simulink model "halfCar_Body"  (R2023b)
settings: Solver=VariableStepAuto  StartTime=0.0  StopTime=10.0  RelTol=1e-3
values from neighbouring files (symbols this model uses):
  a = 1.35    [Parameters.m]
  b = 1.5    [Parameters.m]
  g = 9.81    [Parameters.m]
  I = 650    [Parameters.m]
undefined symbols (not defined in the file or in its folder): Ff, Fr, mb
libraries: simulink x4
settings Model: Creator=crs59  LastModifiedBy=franc
settings DebuggingCC: UnconnectedInputMsg=warning  UnconnectedOutputMsg=warning  UnconnectedLineMsg=warning
settings ModelReferenceCC: EnableRefExpFcnMdlSchedulingChecks=on
settings RTWCC: DLArmComputeVersion=19.05

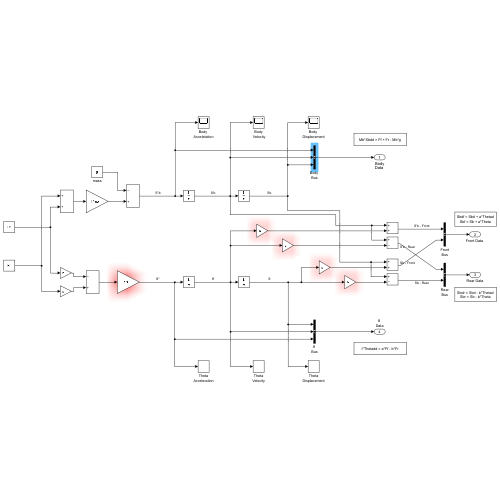
[thumbnail: Simulink's stored preview of the top-level diagram]
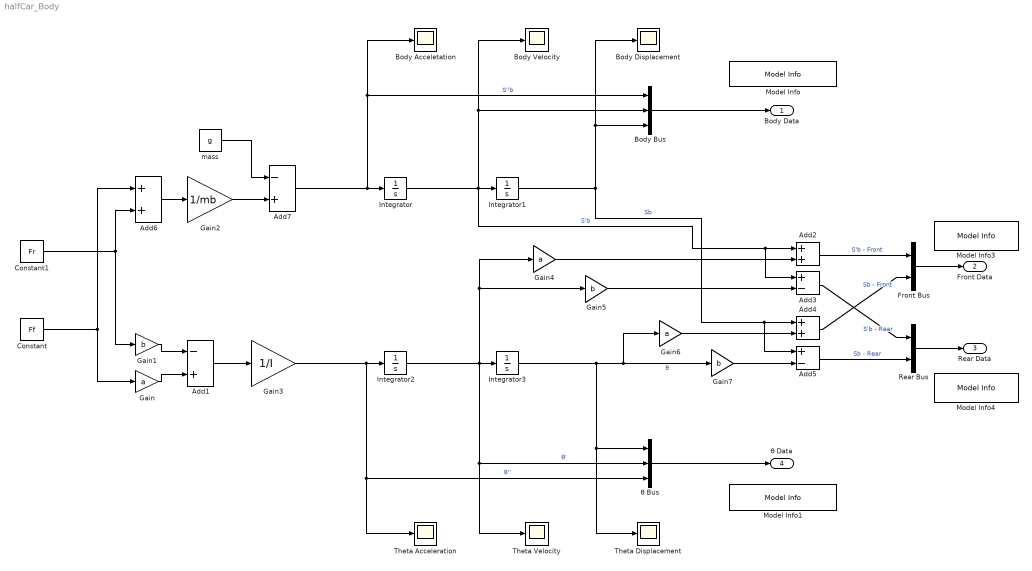
== system halfCar_Body ==
  Add1 : Sum  Inputs=-+
  Add2 : Sum
  Add3 : Sum  Inputs=+-
  Add4 : Sum
  Add5 : Sum  Inputs=+-
  Add6 : Sum
  Add7 : Sum  Inputs=-+
  Body Velocity : Scope
  Body Acceletation : Scope
  Body Bus : BusCreator  Inputs=3
  Body Displacement : Scope
  Constant : Constant  Value=Ff
  Constant1 : Constant  Value=Fr
  Front Bus : BusCreator  Inputs=2
  Gain : Gain  Gain=a
  Gain1 : Gain  Gain=b
  Gain2 : Gain  Gain=1/mb
  Gain3 : Gain  Gain=1/I
  Gain4 : Gain  Gain=a
  Gain5 : Gain  Gain=b
  Gain6 : Gain  Gain=a
  Gain7 : Gain  Gain=b
  Integrator{,1..3} (4 alike) : Integrator
  Model Info : simulink/Model-Wide Utilities/Model Info  Frame=on  DisplayStringWithTags=Mb*Sbdd = Ff + Fr - Mb*g  HorizontalTextAlignment=Center  LeftAlignmentValue=0.5
  Model Info1 : simulink/Model-Wide Utilities/Model Info  Frame=on  DisplayStringWithTags=I*Thetadd = a*Ff - b*Fr  HorizontalTextAlignment=Center  LeftAlignmentValue=0.5
  Model Info3 : simulink/Model-Wide Utilities/Model Info  Frame=on  DisplayStringWithTags=|  HorizontalTextAlignment=Center  LeftAlignmentValue=0.5
      | Sbdf = Sbd + a*Thetad
      | Sbf = Sb + a*Theta
  Model Info4 : simulink/Model-Wide Utilities/Model Info  Frame=on  DisplayStringWithTags=|  HorizontalTextAlignment=Center  LeftAlignmentValue=0.5
      | Sbdr = Sbd - b*Thetad
      | Sbr = Sb - b*Theta
  Rear Bus : BusCreator  Inputs=2
  Theta Acceleration : Scope
  Theta Displacement : Scope
  Theta Velocity : Scope
  mass : Constant  Value=g
  θ Bus : BusCreator  Inputs=3
  "Body Data " : Outport
  "Front Data " : Outport  Port=2
  Rear Data : Outport  Port=3
  θ Data : Outport  Port=4
  wires:
  Integrator2/1 -> θ Bus/2, Theta Velocity/1, Integrator3/1, Gain4/1, Gain5/1  "θ'"
  Add4/1 -> Front Bus/2  "Sb - Front"
  Add3/1 -> Rear Bus/1  "S'b - Rear"
  Add1/1 -> Gain3/1
  Gain7/1 -> Add5/2
  Integrator1/1 -> Body Displacement/1, Body Bus/3, Add4/1, Add5/1  "Sb"
  Gain/1 -> Add1/2
  Gain5/1 -> Add3/2
  mass/1 -> Add7/1
  Gain6/1 -> Add4/2
  Gain1/1 -> Add1/1
  Add5/1 -> Rear Bus/2  "Sb - Rear"
  Rear Bus/1 -> Rear Data/1
  Front Bus/1 -> "Front Data "/1
  Add2/1 -> Front Bus/1  "S'b - Front"
  Gain4/1 -> Add2/2
  Body Bus/1 -> "Body Data "/1
  Constant1/1 -> Add6/2, Gain1/1
  Integrator/1 -> Body Velocity/1, Body Bus/2, Add2/1, Add3/1, Integrator1/1  "S'b"
  θ Bus/1 -> θ Data/1
  Gain3/1 -> θ Bus/3, Theta Acceleration/1, Integrator2/1  "θ''"
  Constant/1 -> Add6/1, Gain/1
  Integrator3/1 -> θ Bus/1, Theta Displacement/1, Gain7/1, Gain6/1  "θ"
  Add6/1 -> Gain2/1
  Gain2/1 -> Add7/2
  Add7/1 -> Body Bus/1, Body Acceletation/1, Integrator/1  "S''b"
